simulink model "model"  (R2021a)
settings: Solver=VariableStepAuto  StartTime=0.0  StopTime=10.0  RelTol=1e-3
libraries: simulink x6, sharedutil x5, aerolibutil x1
(part 1 of 2)
settings Model: Creator=frede  LastModifiedBy=frede
settings DataIOCC: ReturnWorkspaceOutputs=off

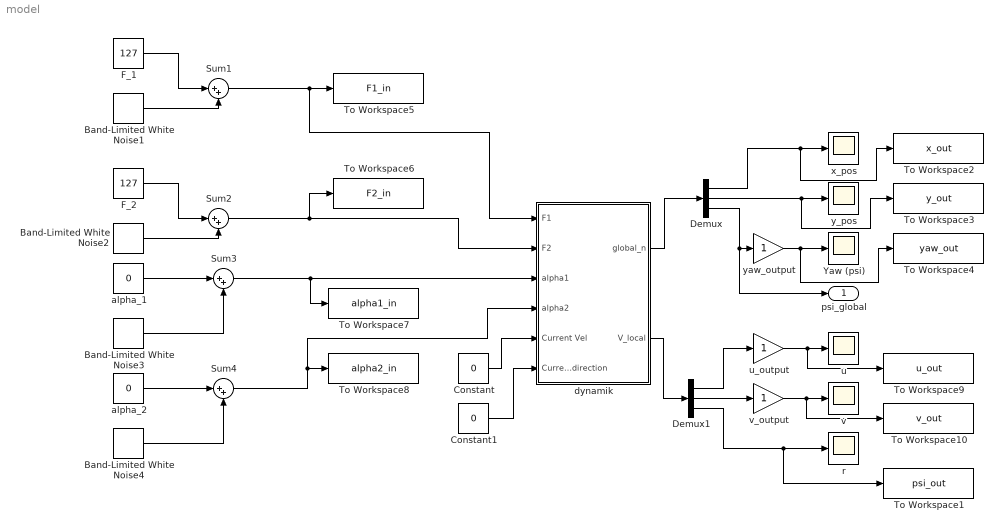
== system model ==
  Band-Limited White Noise{1..4} (4 alike) : simulink/Sources/Band-Limited White Noise  Cov=[0.01]  Ts=0.1  seed=[23341]
  Constant : Constant  Value=0
  Constant1 : Constant  Value=0
  Demux : Demux  Outputs=3
  Demux1 : Demux  Outputs=3
  F_1 : Constant  Value=127
  F_2 : Constant  Value=127
  Sum{1..4} (4 alike) : Sum  Inputs=|++
  To Workspace1 : ToWorkspace  VariableName=psi_out  SaveFormat=Timeseries  SampleTime=-1
  To Workspace10 : ToWorkspace  VariableName=v_out  SaveFormat=Timeseries  SampleTime=-1
  To Workspace2 : ToWorkspace  VariableName=x_out  SaveFormat=Timeseries  SampleTime=-1
  To Workspace3 : ToWorkspace  VariableName=y_out  SaveFormat=Timeseries  SampleTime=-1
  To Workspace4 : ToWorkspace  VariableName=yaw_out  SaveFormat=Timeseries  SampleTime=-1
  To Workspace5 : ToWorkspace  VariableName=F1_in  SaveFormat=Timeseries  SampleTime=-1
  To Workspace6 : ToWorkspace  VariableName=F2_in  SaveFormat=Timeseries  SampleTime=-1
  To Workspace7 : ToWorkspace  VariableName=alpha1_in  SaveFormat=Timeseries  SampleTime=-1
  To Workspace8 : ToWorkspace  VariableName=alpha2_in  SaveFormat=Timeseries  SampleTime=-1
  To Workspace9 : ToWorkspace  VariableName=u_out  SaveFormat=Timeseries  SampleTime=-1
  Yaw (psi) : Scope
  alpha_1 : Constant  Value=0
  alpha_2 : Constant  Value=0
  dynamik : Subsystem
  r : Scope
  u : Scope
  u_output : Gain
  v : Scope
  v_output : Gain
  x_pos : Scope
  y_pos : Scope
  yaw_output : Gain
  psi_global : Outport
  wires:
  Demux/2 -> To Workspace3/1, y_pos/1
  u_output/1 -> To Workspace9/1, u/1
  dynamik/2(V_local) -> Demux1/1
  v_output/1 -> To Workspace10/1, v/1
  Demux1/3 -> To Workspace1/1, r/1
  Demux/3 -> yaw_output/1, psi_global/1
  Demux1/1 -> u_output/1
  yaw_output/1 -> To Workspace4/1, Yaw (psi)/1
  Demux1/2 -> v_output/1
  dynamik/1(global_n) -> Demux/1
  Demux/1 -> To Workspace2/1, x_pos/1
  Constant/1 -> dynamik/5(Current Vel)
  Constant1/1 -> dynamik/6(Current direction)
  Sum3/1 -> To Workspace7/1, dynamik/3(alpha1)
  Sum4/1 -> dynamik/4(alpha2), To Workspace8/1
  Sum2/1 -> dynamik/2(F2), To Workspace6/1
  Sum1/1 -> dynamik/1(F1), To Workspace5/1
  F_1/1 -> Sum1/1
  Band-Limited White Noise1/1 -> Sum1/2
  F_2/1 -> Sum2/1
  Band-Limited White Noise2/1 -> Sum2/2
  alpha_1/1 -> Sum3/1
  Band-Limited White Noise3/1 -> Sum3/2
  Band-Limited White Noise4/1 -> Sum4/2
  alpha_2/1 -> Sum4/1

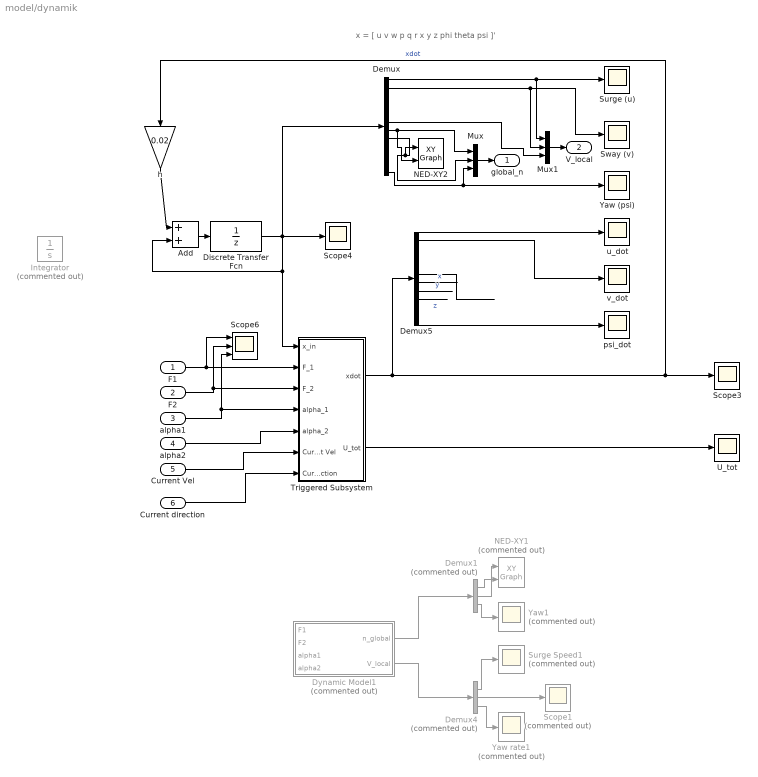
== system model/dynamik ==
  note: x = [ u v w p q r x y z phi theta psi ]'
  F1 : Inport
  F2 : Inport  Port=2
  alpha1 : Inport  Port=3
  alpha2 : Inport  Port=4
  Current Vel : Inport  Port=5
  Current direction : Inport  Port=6
  Add : Sum
  Demux : Demux  Outputs=12
  Demux1 : Demux  Commented=on  Outputs=3
  Demux4 : Demux  Commented=on  Outputs=3
  Demux5 : Demux  Outputs=12
  Discrete Transfer Fcn : DiscreteTransferFcn  Denominator=[ 1 0]  SampleTime=0.02
  Dynamic Model1 : Subsystem  Commented=on
  Integrator : Integrator  Commented=on
  Mux : Mux  Inputs=3
  Mux1 : Mux  Inputs=3
  NED-XY1 : simulink/Sinks/XY Graph  Commented=on  xmin=-1000  xmax=1000  ymin=-1000  ymax=1000  st=-1
  NED-XY2 : simulink/Sinks/XY Graph  xmin=-1000  xmax=1000  ymin=-1000  ymax=1000  st=-1
  Scope1 : Scope  Commented=on
  Scope3 : Scope
  Scope4 : Scope
  Scope6 : Scope  NumInputPorts=3
  Surge (u) : Scope
  Surge Speed1 : Scope  Commented=on
  Sway (v) : Scope
  Triggered Subsystem : Subsystem  TreatAsAtomicUnit=on
  U_tot : Scope
  Yaw (psi) : Scope
  Yaw rate1 : Scope  Commented=on
  Yaw1 : Scope  Commented=on
  h : Gain  Gain=0.02
  psi_dot : Scope
  u_dot : Scope
  v_dot : Scope
  global_n : Outport
  V_local : Outport  Port=2
  wires:
  Demux1/3 -> Yaw1/1
  Demux4/3 -> Yaw rate1/1
  Demux1/2 -> NED-XY1/1
  Demux4/2 -> Scope1/1
  Demux1/1 -> NED-XY1/2
  Demux4/1 -> Surge Speed1/1
  Dynamic Model1/1(n_global) -> Demux1/1
  Dynamic Model1/2(V_local) -> Demux4/1
  F1/1 -> Scope6/1, Triggered Subsystem/2(F_1)
  F2/1 -> Scope6/2, Triggered Subsystem/3(F_2)
  alpha1/1 -> Scope6/3, Triggered Subsystem/4(alpha_1)
  alpha2/1 -> Triggered Subsystem/5(alpha_2)
  h/1 -> Add/1
  Add/1 -> Discrete Transfer Fcn/1
  Triggered Subsystem/1(xdot) -> Demux5/1, Scope3/1, h/1  "xdot"
  Triggered Subsystem/2(U_tot) -> U_tot/1
  Demux/8 -> Mux/2, NED-XY2/1
  Demux/7 -> NED-XY2/2, Mux/1
  Discrete Transfer Fcn/1 -> Scope4/1, Demux/1, Add/2, Triggered Subsystem/1(x_in)
  Demux/1 -> Surge (u)/1, Mux1/1
  Demux/12 -> Mux/3, Yaw (psi)/1
  Demux/2 -> Mux1/2, Sway (v)/1
  Mux/1 -> global_n/1
  Demux5/12 -> psi_dot/1
  Demux5/2 -> v_dot/1
  Demux5/1 -> u_dot/1
  Demux5/9 -> ?  "z"
  Demux5/7 -> ?  "x"
  Demux5/8 -> ?  "y"
  Mux1/1 -> V_local/1
  Demux5/6 -> ?
  Demux/6 -> Mux1/3
  Current Vel/1 -> Triggered Subsystem/6(Current Vel)
  Current direction/1 -> Triggered Subsystem/7(Current Direction)

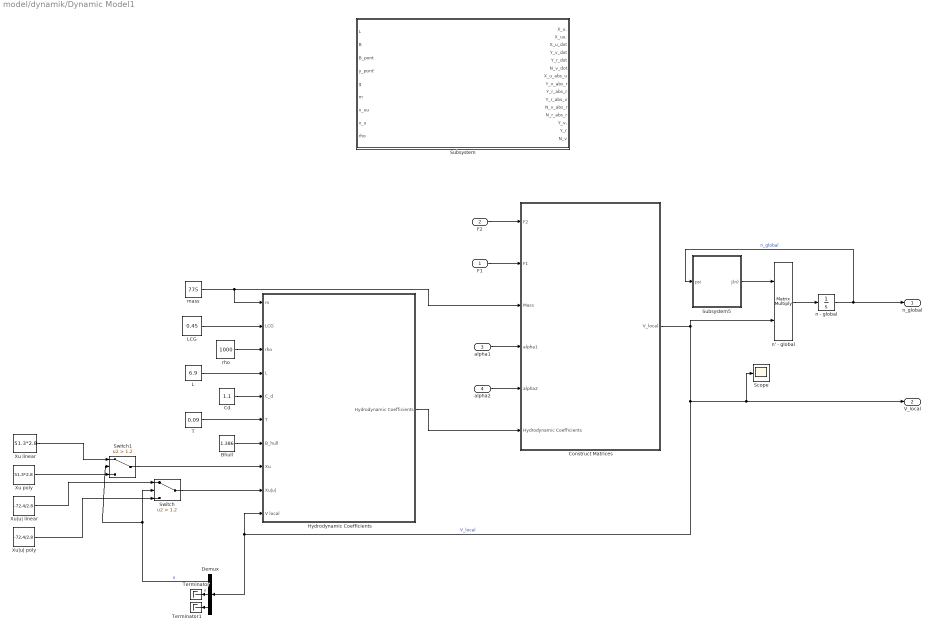
== system model/dynamik/Dynamic Model1 ==
  F1 : Inport
  F2 : Inport  Port=2
  alpha1 : Inport  Port=3
  alpha2 : Inport  Port=4
  "Bhull " : Constant  Value=1.386
  Cd : Constant  Value=1.1
  Construct Matrices : Subsystem
  Demux : Demux  Outputs=3
  Hydrodynamic Coefficients : Subsystem
  L : Constant  Value=6.9
  LCG : Constant  Value=0.45
  Scope : Scope
  Subsystem : Subsystem
  Subsystem5 : Subsystem
  Switch : Switch  Criteria=u2 > Threshold  Threshold=1.2
  Switch1 : Switch  Criteria=u2 > Threshold  Threshold=1.2
  T : Constant  Value=0.09
  Terminator : Terminator
  Terminator1 : Terminator
  Xu linear : Constant  Value=51.3*2.8
  Xu poly : Constant  Value=51.3*2.8
  Xu|u| linear : Constant  Value=-72.4/2.8
  Xu|u| poly : Constant  Value=-72.4/2.8
  mass : Constant  Value=775
  n - global : Integrator  InitialCondition=[0 0 0]
  n' - global : Product  Multiplication=Matrix(*)
  rho : Constant  Value=1000
  n_global : Outport  VectorParamsAs1DForOutWhenUnconnected=off
  V_local : Outport  Port=2  VectorParamsAs1DForOutWhenUnconnected=off
  wires:
  n - global/1 -> Subsystem5/1(psi), n_global/1  "n_global"
  Cd/1 -> Hydrodynamic Coefficients/5(C_d)
  Construct Matrices/1(V_local) -> n' - global/2, Demux/1, Hydrodynamic Coefficients/10(V local), Scope/1, V_local/1  "V_local"
  n' - global/1 -> n - global/1
  Subsystem5/1(J(n)) -> n' - global/1
  rho/1 -> Hydrodynamic Coefficients/3(rho)
  L/1 -> Hydrodynamic Coefficients/4(L)
  F2/1 -> Construct Matrices/1(F2)
  F1/1 -> Construct Matrices/2(F1)
  mass/1 -> Hydrodynamic Coefficients/1(m), Construct Matrices/3("Mass ")
  Hydrodynamic Coefficients/1("Hydrodynamic Coefficients ") -> Construct Matrices/6(Hydrodynamic Coefficients)
  T/1 -> Hydrodynamic Coefficients/6(T)
  "Bhull "/1 -> Hydrodynamic Coefficients/7(B_hull)
  Switch/1 -> Hydrodynamic Coefficients/9(Xu|u|)
  LCG/1 -> Hydrodynamic Coefficients/2(LCG)
  Demux/1 -> Switch1/2, Switch/2  "u"
  Xu|u| poly/1 -> Switch/3
  Xu|u| linear/1 -> Switch/1
  Switch1/1 -> Hydrodynamic Coefficients/8(Xu)
  Xu poly/1 -> Switch1/3
  Xu linear/1 -> Switch1/1
  Demux/3 -> Terminator1/1
  Demux/2 -> Terminator/1  "v"
  alpha1/1 -> Construct Matrices/4(alpha1)
  alpha2/1 -> Construct Matrices/5(alpha2)

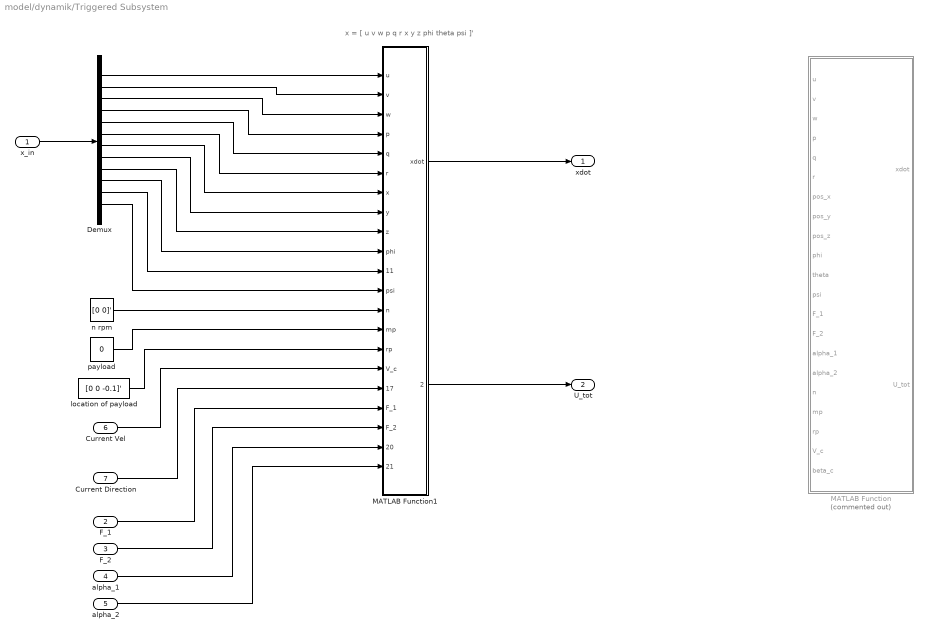
== system model/dynamik/Triggered Subsystem ==
  note: x = [ u v w p q r x y z phi theta psi ]'
  x_in : Inport
  F_1 : Inport  Port=2
  F_2 : Inport  Port=3
  alpha_1 : Inport  Port=4
  alpha_2 : Inport  Port=5
  Current Vel : Inport  Port=6
  Current Direction : Inport  Port=7
  Demux : Demux  Outputs=12
  MATLAB Function : MATLAB Function  Commented=on  TreatAsAtomicUnit=on
  MATLAB Function1 : MATLAB Function  TreatAsAtomicUnit=on
  location of payload : Constant  Value=[0 0 -0.1]'
  n rpm : Constant  Value=[0 0]'
  payload : Constant  Value=0
  xdot : Outport
  U_tot : Outport  Port=2
  wires:
  F_1/1 -> MATLAB Function1/18(F_1)
  F_2/1 -> MATLAB Function1/19(F_2)
  alpha_1/1 -> MATLAB Function1/20(alpha_1)
  alpha_2/1 -> MATLAB Function1/21(alpha_2)
  location of payload/1 -> MATLAB Function1/15(rp)
  payload/1 -> MATLAB Function1/14(mp)
  Current Vel/1 -> MATLAB Function1/16(V_c)
  Current Direction/1 -> MATLAB Function1/17(beta_c)
  n rpm/1 -> MATLAB Function1/13(n)
  x_in/1 -> Demux/1
  MATLAB Function1/2(U_tot) -> U_tot/1
  MATLAB Function1/1(xdot) -> xdot/1
  Demux/1 -> MATLAB Function1/1(u)
  Demux/2 -> MATLAB Function1/2(v)
  Demux/3 -> MATLAB Function1/3(w)
  Demux/4 -> MATLAB Function1/4(p)
  Demux/5 -> MATLAB Function1/5(q)
  Demux/6 -> MATLAB Function1/6(r)
  Demux/7 -> MATLAB Function1/7(x)
  Demux/8 -> MATLAB Function1/8(y)
  Demux/9 -> MATLAB Function1/9(z)
  Demux/10 -> MATLAB Function1/10(phi)
  Demux/11 -> MATLAB Function1/11(theta)
  Demux/12 -> MATLAB Function1/12(psi)

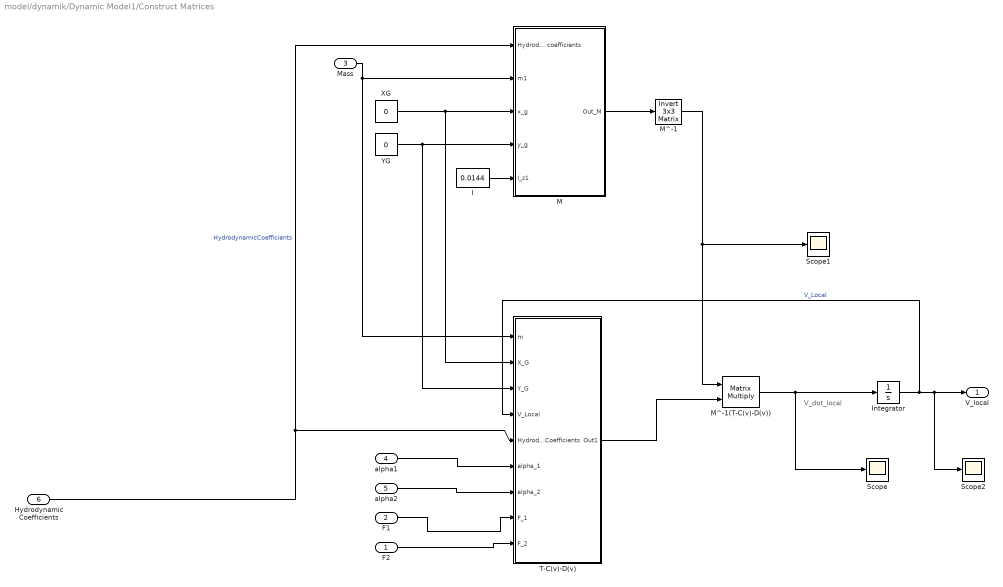
== system model/dynamik/Dynamic Model1/Construct Matrices ==
  note: V_dot_local
  F2 : Inport
  F1 : Inport  Port=2
  "Mass " : Inport  Port=3
  alpha1 : Inport  Port=4
  alpha2 : Inport  Port=5
  Hydrodynamic Coefficients : Inport  Port=6
  I : Constant  Value=0.0144
  Integrator : Integrator  InitialCondition=[0 0 0]
  M : Subsystem
  M^-1 : aerolibutil/Invert  3x3 Matrix
  M^-1(T-C(v)-D(v)) : Product  Multiplication=Matrix(*)
  Scope : Scope
  Scope1 : Scope
  Scope2 : Scope
  T-C(v)-D(v) : Subsystem
  XG : Constant  Value=0
  YG : Constant  Value=0
  V_local : Outport  VectorParamsAs1DForOutWhenUnconnected=off
  wires:
  Integrator/1 -> Scope2/1, V_local/1, T-C(v)-D(v)/4(V_Local)  "V_Local"
  M^-1(T-C(v)-D(v))/1 -> Scope/1, Integrator/1
  M/1(Out_M) -> M^-1/1
  Hydrodynamic Coefficients/1 -> M/1(Hydrodynamic coefficients), T-C(v)-D(v)/5(HydrodynamicCoefficients)  "HydrodynamicCoefficients"
  YG/1 -> M/4(y_g), T-C(v)-D(v)/3(Y_G)
  "Mass "/1 -> T-C(v)-D(v)/1(m), M/2(m1)
  XG/1 -> M/3(x_g), T-C(v)-D(v)/2(X_G)
  F1/1 -> T-C(v)-D(v)/8(F_1)
  F2/1 -> T-C(v)-D(v)/9(F_2)
  T-C(v)-D(v)/1(Out1) -> M^-1(T-C(v)-D(v))/2
  I/1 -> M/5(I_z1)
  alpha1/1 -> T-C(v)-D(v)/6(alpha_1)
  alpha2/1 -> T-C(v)-D(v)/7(alpha_2)
  M^-1/1 -> Scope1/1, M^-1(T-C(v)-D(v))/1

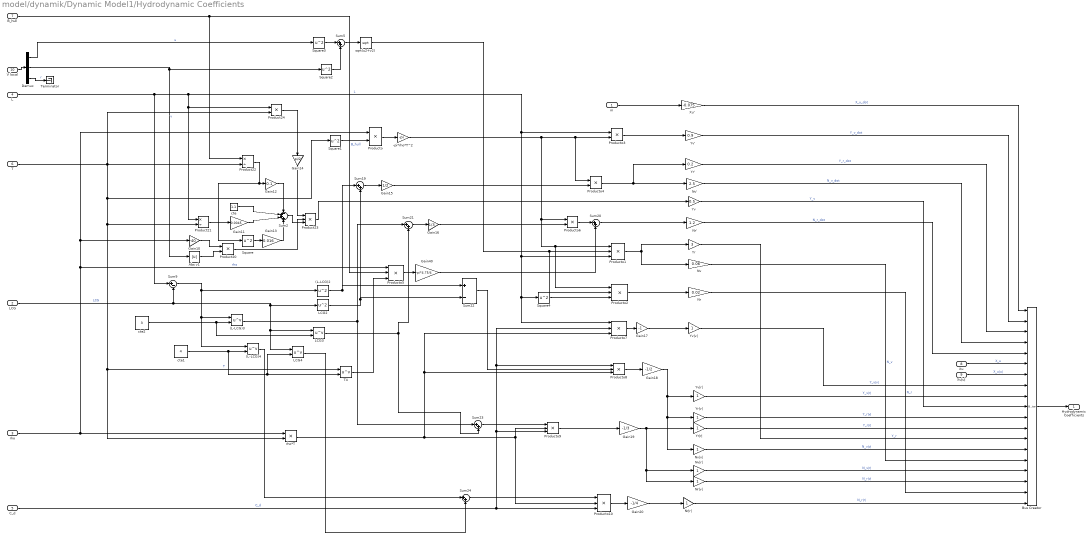
== system model/dynamik/Dynamic Model1/Hydrodynamic Coefficients ==
  m : Inport
  LCG : Inport  Port=2
  rho : Inport  Port=3
  L : Inport  Port=4
  C_d : Inport  Port=5
  T : Inport  Port=6
  B_hull : Inport  Port=7
  Xu : Inport  Port=8
  Xu|u| : Inport  Port=9
  V local : Inport  Port=10
  (L-LCG)2 : Math  Operator=square  SignedPower=on  SaturateOnIntegerOverflow=on
  (L-LCG)3 : Math  Operator=pow  SignedPower=on  SaturateOnIntegerOverflow=on
  (L-LCG)4 : Math  Operator=pow  SignedPower=on  SaturateOnIntegerOverflow=on
  -pi*rho*T^2 : Gain  Gain=-pi
  Abs v1 : Abs
  Bus Creator : BusCreator  Inputs=19
  Demux : Demux  Outputs=3
  Gain10 : Gain  Gain=-40
  Gain11 : Gain  Gain=0.0045
  Gain12 : Gain  Gain=0.1
  Gain13 : Gain  Gain=0.016
  Gain14 : Gain  Gain=pi/2
  Gain15 : Gain  Gain=1/2
  Gain16 : Gain  Gain=1/3
  Gain17 : Gain  Gain=-1
  Gain18 : Gain  Gain=-1/2
  Gain19 : Gain  Gain=-1/3
  Gain20 : Gain  Gain=-1/4
  Gain40 : Gain  Gain=-pi*4.75/4
  LCG2 : Math  Operator=square  SignedPower=on  SaturateOnIntegerOverflow=on
  LCG3 : Math  Operator=pow  SignedPower=on  SaturateOnIntegerOverflow=on
  LCG4 : Math  Operator=pow  SignedPower=on  SaturateOnIntegerOverflow=on
  Nr : Gain  Gain=0.02
  Nr' : Gain  Gain=1.2
  Nr|r| : Gain
  Nr|v| : Gain
  Nv : Gain  Gain=0.06
  Nv' : Gain  Gain=2.5
  Nv|r| : Gain
  Nv|v| : Gain
  Product20 : Product
  Product21 : Product  Inputs=*/
  Product22 : Product  Inputs=*/
  Product23 : Product  Inputs=3
  Product24 : Product
  Producto{,3..4,6} (4 alike) : Product
  Producto{1..2,5,7..10} (7 alike) : Product  Inputs=3
  Square{,1..4} (5 alike) : Math  Operator=square  SignedPower=on  SaturateOnIntegerOverflow=on
  Sum{5,19..21,23..24} (6 alike) : Sum  Inputs=|++
  Sum2 : Sum  Inputs=-+++
  Sum22 : Sum  Inputs=|+-
  Sum9 : Sum  Inputs=|+-
  T4 : Math  Operator=pow  SignedPower=on  SaturateOnIntegerOverflow=on
  Terminator : Terminator
  Xu' : Gain  Gain=-0.075
  Yr : Gain  Gain=3
  Yr' : Gain  Gain=0.2
  Yr|r| : Gain
  Yr|v| : Gain
  Yv : Gain  Gain=0.5
  Yv' : Gain  Gain=0.9
  Yv|r| : Gain
  Yv|v| : Gain
  cte : Constant  Value=1.1
  cte1 : Constant  Value=4
  cte2 : Constant  Value=3
  rho*T : Product
  sqrt(u2+v2) : Sqrt  SaturateOnIntegerOverflow=on
  "Hydrodynamic Coefficients " : Outport  VectorParamsAs1DForOutWhenUnconnected=off
  wires:
  m/1 -> Xu'/1
  Nv'/1 -> Bus Creator/4  "N_v_dot"
  Xu'/1 -> Bus Creator/1  "X_u_dot"
  Square/1 -> Gain13/1
  Gain14/1 -> Product23/1
  Product24/1 -> Gain14/1
  Sum9/1 -> (L-LCG)3/1, (L-LCG)4/1, (L-LCG)2/1
  Square4/1 -> Producto2/3
  sqrt(u2+v2)/1 -> Producto2/2, Producto1/2
  Product20/1 -> Product23/2
  Gain13/1 -> Sum2/4
  B_hull/1 -> Producto5/2, Product22/1  "B_hull"
  Square2/1 -> Sum5/2
  Sum20/1 -> Nr'/1
  Gain12/1 -> Sum2/1
  Sum21/1 -> Gain16/1
  LCG4/1 -> Sum24/2
  Sum24/1 -> Producto10/1
  (L-LCG)4/1 -> Sum24/1
  Sum2/1 -> Product23/3
  Producto10/1 -> Gain20/1
  (L-LCG)3/1 -> Sum21/1, Sum23/1
  Producto6/1 -> Sum20/1
  Gain19/1 -> Yr|r|/1, Nr|v|/1, Nv|r|/1
  Gain16/1 -> Producto6/2
  Sum22/1 -> Producto8/2
  Producto3/1 -> Yv'/1
  Gain10/1 -> Product20/1
  cte1/1 -> LCG4/2, T4/2, (L-LCG)4/2
  cte2/1 -> (L-LCG)3/2, LCG3/2
  Product23/1 -> Yv/1
  cte/1 -> Sum2/2
  Producto8/1 -> Gain18/1
  Sum23/1 -> Producto9/1
  Gain20/1 -> Nr|r|/1
  Gain18/1 -> Nv|v|/1, Yr|v|/1, Yv|r|/1
  Yr'/1 -> Bus Creator/3  "Y_r_dot"
  Producto7/1 -> Gain17/1
  Producto9/1 -> Gain19/1
  Gain11/1 -> Sum2/3
  Square1/1 -> Producto/2
  Producto2/1 -> Nr/1
  LCG3/1 -> Sum21/2, Sum23/2
  T4/1 -> Producto5/3
  Gain40/1 -> Sum20/2
  Producto4/1 -> Yr'/1, Nv'/1
  Sum19/1 -> Gain15/1
  Square3/1 -> Sum5/1
  Sum5/1 -> sqrt(u2+v2)/1
  rho/1 -> Producto/1, Gain10/1, Producto5/1, rho*T/1  "rho"
  Abs v1/1 -> Product20/2
  Product21/1 -> Gain11/1
  Gain17/1 -> Yv|v|/1
  (L-LCG)2/1 -> Sum19/1, Sum22/1
  Producto1/1 -> Nv/1, Yr/1
  Product22/1 -> Square/1, Gain12/1
  LCG2/1 -> Sum19/2, Sum22/2
  LCG/1 -> Sum9/2, LCG2/1, LCG3/1, LCG4/1  "LCG"
  Producto/1 -> -pi*rho*T^2/1
  -pi*rho*T^2/1 -> Producto4/1, Producto3/2, Producto2/1, Producto1/1, Producto6/1
  Producto5/1 -> Gain40/1
  Gain15/1 -> Producto4/2
  rho*T/1 -> Producto9/2, Producto10/2, Producto7/3, Producto8/3
  T/1 -> Product21/2, rho*T/2, T4/1, Square1/1, Product22/2, Product24/2  "T"
  L/1 -> Producto7/1, Square4/1, Producto1/3, Producto3/1, Product21/1, Product24/1, Sum9/1  "L"
  C_d/1 -> Producto7/2, Producto8/1, Producto9/3, Producto10/3  "C_d"
  Nv/1 -> Bus Creator/15  "N_v"
  Yv|v|/1 -> Bus Creator/8  "Y_v|v|"
  Yr|r|/1 -> Bus Creator/12  "Y_r|r|"
  Yv/1 -> Bus Creator/10  "Y_v"
  Nv|v|/1 -> Bus Creator/14  "N_v|v|"
  Yr|v|/1 -> Bus Creator/11  "Y_r|v|"
  Nv|r|/1 -> Bus Creator/16  "N_v|r|"
  Yr/1 -> Bus Creator/13  "Y_r"
  Nr|r|/1 -> Bus Creator/19  "N_r|r|"
  Nr/1 -> Bus Creator/18  "N_r"
  Xu|u|/1 -> Bus Creator/7  "X_u|u|"
  Yv|r|/1 -> Bus Creator/9  "Y_v|r|"
  Nr|v|/1 -> Bus Creator/17  "N_r|v|"
  Xu/1 -> Bus Creator/6  "X_u"
  Bus Creator/1 -> "Hydrodynamic Coefficients "/1
  Nr'/1 -> Bus Creator/5  "N_r_dot"
  Yv'/1 -> Bus Creator/2  "Y_v_dot"
  Demux/1 -> Square3/1  "u"
  V local/1 -> Demux/1
  Demux/2 -> Abs v1/1, Square2/1  "v"
  Demux/3 -> Terminator/1  "r"

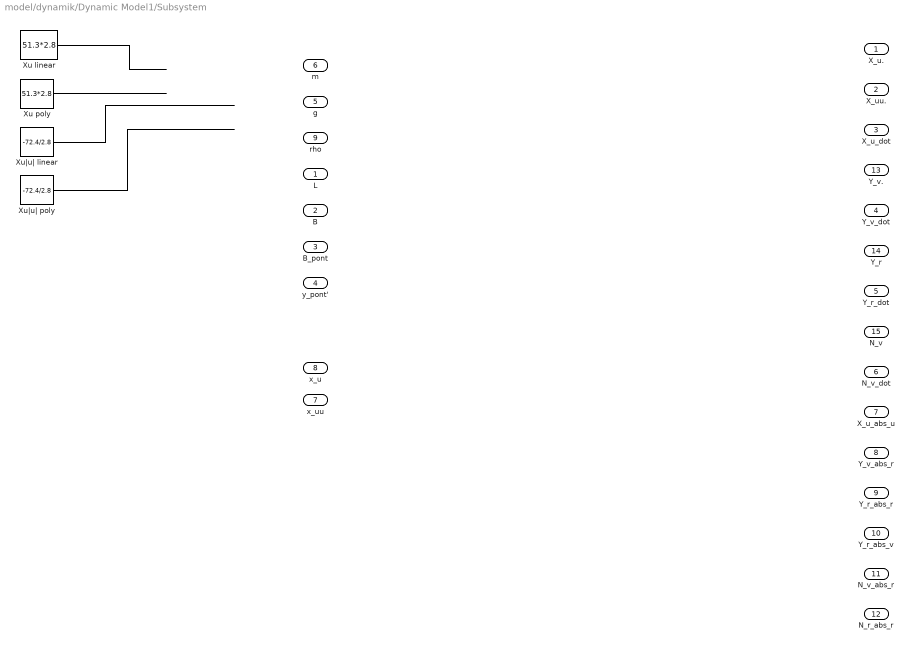
== system model/dynamik/Dynamic Model1/Subsystem ==
  L : Inport
  B : Inport  Port=2
  B_pont : Inport  Port=3
  y_pont' : Inport  Port=4
  g : Inport  Port=5
  m : Inport  Port=6
  x_uu : Inport  Port=7
  x_u : Inport  Port=8
  rho : Inport  Port=9
  Xu linear : Constant  Value=51.3*2.8
  Xu poly : Constant  Value=51.3*2.8
  Xu|u| linear : Constant  Value=-72.4/2.8
  Xu|u| poly : Constant  Value=-72.4/2.8
  X_u. : Outport
  X_uu. : Outport  Port=2
  X_u_dot : Outport  Port=3
  Y_v_dot : Outport  Port=4
  Y_r_dot : Outport  Port=5
  N_v_dot : Outport  Port=6
  X_u_abs_u : Outport  Port=7
  Y_v_abs_r : Outport  Port=8
  Y_r_abs_r : Outport  Port=9
  Y_r_abs_v : Outport  Port=10
  N_v_abs_r : Outport  Port=11
  N_r_abs_r : Outport  Port=12
  Y_v. : Outport  Port=13
  Y_r : Outport  Port=14
  N_v : Outport  Port=15
  wires:
  Xu|u| linear/1 -> ?
  Xu|u| poly/1 -> ?
  Xu poly/1 -> ?
  Xu linear/1 -> ?

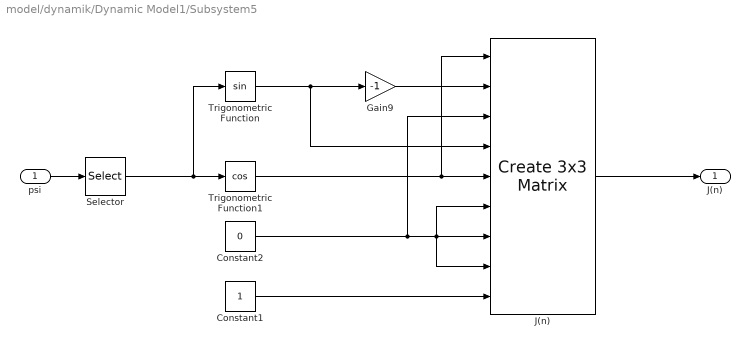
== system model/dynamik/Dynamic Model1/Subsystem5 ==
  psi : Inport
  " J(n)" : sharedutil/Create 3x3 Matrix  aMode=aMode
      settings: SourceProductBaseCode=AE,PW,DR,MT,UV,VE
  Constant1 : Constant
  Constant2 : Constant  Value=0
  Gain9 : Gain  Gain=-1
  Selector : Selector  InputPortWidth=3  IndexOptions=Index vector (dialog)  Indices=3  OutputSizes=1
  Trigonometric Function : Trigonometry
  Trigonometric Function1 : Trigonometry  Operator=cos
  J(n) : Outport  VectorParamsAs1DForOutWhenUnconnected=off
  wires:
  Gain9/1 -> " J(n)"/2
  Trigonometric Function1/1 -> " J(n)"/5, " J(n)"/1
  Trigonometric Function/1 -> " J(n)"/4, Gain9/1
  Constant1/1 -> " J(n)"/9
  psi/1 -> Selector/1
  " J(n)"/1 -> J(n)/1
  Constant2/1 -> " J(n)"/8, " J(n)"/7, " J(n)"/6, " J(n)"/3
  Selector/1 -> Trigonometric Function1/1, Trigonometric Function/1

== system model/dynamik/Dynamic Model1/Construct Matrices/M ==
  Hydrodynamic coefficients : Inport
  m1 : Inport  Port=2
  x_g : Inport  Port=3
  y_g : Inport  Port=4
  I_z1 : Inport  Port=5
  Bus Selector : BusSelector  OutputSignals=X_u_dot,Y_r_dot,N_v_dot,Y_v_dot,N_r_dot
  M-matrice : MATLAB Function  TreatAsAtomicUnit=on
  Out_M : Outport
  wires:
  Hydrodynamic coefficients/1 -> Bus Selector/1
  m1/1 -> M-matrice/1(m)
  I_z1/1 -> M-matrice/4(I_z)
  y_g/1 -> M-matrice/3(y_g)
  x_g/1 -> M-matrice/2(x_g)
  M-matrice/1(M_out) -> Out_M/1
  Bus Selector/1 -> M-matrice/5(Xu_dot)  "<X_u_dot>"
  Bus Selector/2 -> M-matrice/7(Yr_dot)  "<Y_r_dot>"
  Bus Selector/4 -> M-matrice/6(Yv_dot)  "<Y_v_dot>"
  Bus Selector/5 -> M-matrice/8(Nr_dot)  "<N_r_dot>"
  Bus Selector/3 -> M-matrice/9(Nv_dot)  "<N_v_dot>"

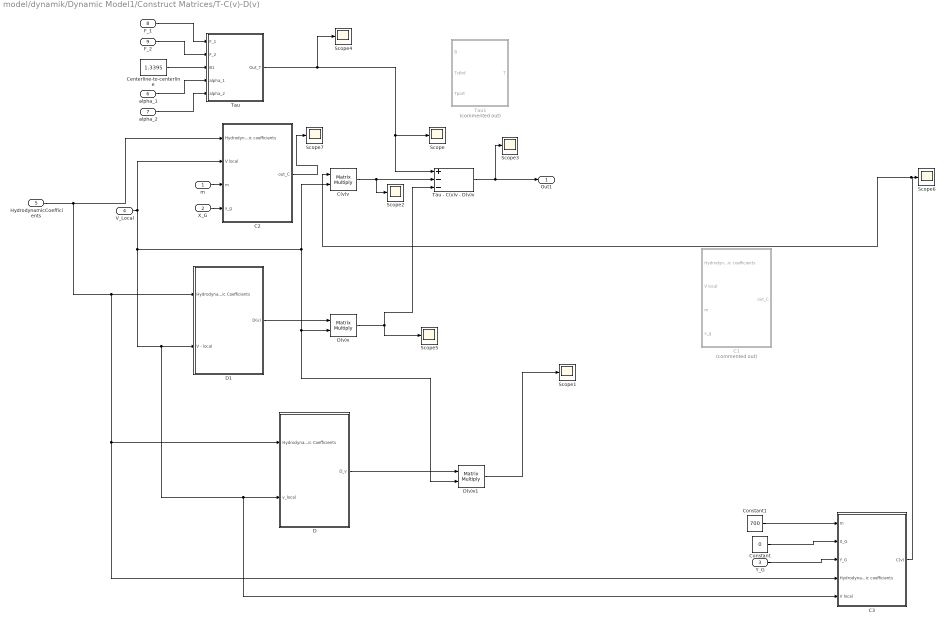
== system model/dynamik/Dynamic Model1/Construct Matrices/T-C(v)-D(v) ==
  m : Inport
  X_G : Inport  Port=2
  Y_G : Inport  Port=3
  V_Local : Inport  Port=4
  HydrodynamicCoefficients : Inport  Port=5
  alpha_1 : Inport  Port=6
  alpha_2 : Inport  Port=7
  F_1 : Inport  Port=8
  F_2 : Inport  Port=9
  C(v)v : Product  Multiplication=Matrix(*)
  C1 : Subsystem  Commented=on
  C2 : Subsystem
  C3 : Subsystem
  Centerline-to-centerline : Constant  Value=1.3395
  Constant : Constant  Value=0
  Constant1 : Constant  Value=700
  D : Subsystem
  D(v)v : Product  Multiplication=Matrix(*)
  D(v)v1 : Product  Multiplication=Matrix(*)
  D1 : Subsystem
  Scope{,1..7} (8 alike) : Scope
  Tau : Subsystem
  Tau - C(v)v - D(v)v : Sum  Inputs=+--
  Tau1 : Subsystem  Commented=on
  Out1 : Outport  VectorParamsAs1DForOutWhenUnconnected=off
  wires:
  V_Local/1 -> C2/2(V local), C3/5(V local), D/2(v_local), D1/2(V - local), D(v)v1/2, D(v)v/2, C(v)v/2
  Tau - C(v)v - D(v)v/1 -> Scope3/1, Out1/1
  HydrodynamicCoefficients/1 -> C2/1(Hydrodynamic coefficients), D/1(Hydrodynamic Coefficients), C3/4(Hydrodynamic coefficients), D1/1(Hydrodynamic Coefficients)
  Centerline-to-centerline/1 -> Tau/3(B1)
  F_2/1 -> Tau/2(F_2)
  F_1/1 -> Tau/1(F_1)
  m/1 -> C2/3(m)
  X_G/1 -> C2/4(x_g)
  Y_G/1 -> C3/3(Y_G)
  C2/1(out_C) -> Scope7/1
  D1/1(D(v)) -> D(v)v/1
  C(v)v/1 -> Scope2/1, Tau - C(v)v - D(v)v/2
  alpha_1/1 -> Tau/4(alpha_1)
  alpha_2/1 -> Tau/5(alpha_2)
  D/1(D_v) -> D(v)v1/1
  D(v)v/1 -> Tau - C(v)v - D(v)v/3, Scope5/1
  D(v)v1/1 -> Scope1/1
  Tau/1(Out_T) -> Scope4/1, Scope/1, Tau - C(v)v - D(v)v/1
  Constant/1 -> C3/2(X_G)
  Constant1/1 -> C3/1(m)
  C3/1(C(v)) -> C(v)v/1, Scope6/1

== system model/dynamik/Dynamic Model1/Construct Matrices/T-C(v)-D(v)/C1 ==
  Hydrodynamic coefficients : Inport
  V local : Inport  Port=2
  m : Inport  Port=3
  x_g : Inport  Port=4
  Demux : Demux  Outputs=19
  Demux1 : Demux  Outputs=3
  MATLAB Function : MATLAB Function  TreatAsAtomicUnit=on
  out_C : Outport
  wires:
  Hydrodynamic coefficients/1 -> Demux/1
  V local/1 -> Demux1/1
  MATLAB Function/1(y) -> out_C/1
  Demux1/1 -> MATLAB Function/2(u)  "u"
  Demux1/2 -> MATLAB Function/1(v)  "v"
  Demux1/3 -> MATLAB Function/3(r)  "r"
  Demux/1 -> MATLAB Function/6(Xu_dot)
  Demux/2 -> MATLAB Function/7(Yv_dot)
  Demux/3 -> MATLAB Function/8(Yr_dot)
  x_g/1 -> MATLAB Function/5(x_g)
  m/1 -> MATLAB Function/4(m)

== system model/dynamik/Dynamic Model1/Construct Matrices/T-C(v)-D(v)/C2 ==
  Hydrodynamic coefficients : Inport
  V local : Inport  Port=2
  m : Inport  Port=3
  x_g : Inport  Port=4
  Demux : Demux  Outputs=19
  Demux1 : Demux  Outputs=3
  MATLAB Function : MATLAB Function  TreatAsAtomicUnit=on
  out_C : Outport
  wires:
  Hydrodynamic coefficients/1 -> Demux/1
  V local/1 -> Demux1/1
  MATLAB Function/1(y) -> out_C/1
  Demux1/1 -> MATLAB Function/2(u)  "u"
  Demux1/2 -> MATLAB Function/1(v)  "v"
  Demux1/3 -> MATLAB Function/3(r)  "r"
  Demux/1 -> MATLAB Function/6(Xu_dot)
  Demux/2 -> MATLAB Function/7(Yv_dot)
  Demux/3 -> MATLAB Function/8(Yr_dot)
  x_g/1 -> MATLAB Function/5(x_g)
  m/1 -> MATLAB Function/4(m)

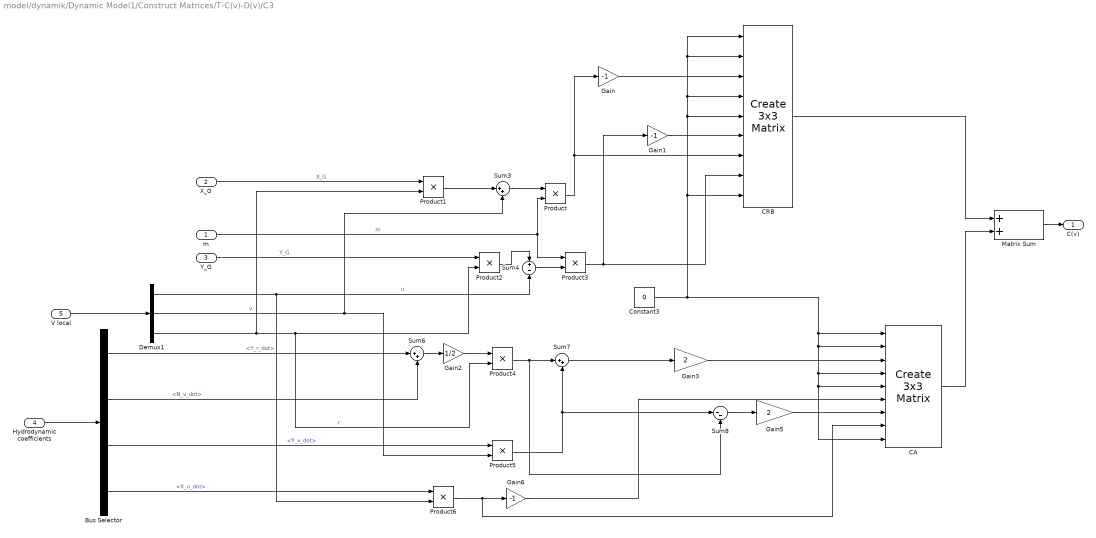
== system model/dynamik/Dynamic Model1/Construct Matrices/T-C(v)-D(v)/C3 ==
  m : Inport
  X_G : Inport  Port=2
  Y_G : Inport  Port=3
  Hydrodynamic coefficients : Inport  Port=4
  V local : Inport  Port=5
  " CRB" : sharedutil/Create 3x3 Matrix  aMode=aMode
      settings: SourceProductBaseCode=AE,PW,DR,MT,UV,VE
  Bus Selector : BusSelector  OutputSignals=Y_r_dot,N_v_dot,Y_v_dot,X_u_dot
  CA : sharedutil/Create 3x3 Matrix  aMode=aMode
      settings: SourceProductBaseCode=AE,PW,DR,MT,UV,VE
  Constant3 : Constant  Value=0
  Demux1 : Demux  Outputs=3
  Gain : Gain  Gain=-1
  Gain1 : Gain  Gain=-1
  Gain2 : Gain  Gain=1/2
  Gain3 : Gain  Gain=2
  Gain5 : Gain  Gain=2
  Gain6 : Gain  Gain=-1
  Matrix Sum : Sum
  Product{,1..6} (7 alike) : Product
  Sum3 : Sum  Inputs=|++
  Sum4 : Sum  Inputs=+-
  Sum6 : Sum  Inputs=|++
  Sum7 : Sum  Inputs=|++
  Sum8 : Sum  Inputs=|--
  C(v) : Outport  VectorParamsAs1DForOutWhenUnconnected=off
  wires:
  Bus Selector/1 -> Sum6/1  "<Y_r_dot>"
  Demux1/3 -> Product1/2, Product2/2, Product4/2  "r"
  Gain2/1 -> Product4/1
  CA/1 -> Matrix Sum/2
  Gain/1 -> " CRB"/3
  Bus Selector/2 -> Sum6/2  "<N_v_dot>"
  Sum3/1 -> Product/1
  Sum8/1 -> Gain5/1
  Product2/1 -> Sum4/1
  Sum6/1 -> Gain2/1
  Product5/1 -> Sum7/2, Sum8/1
  Gain1/1 -> " CRB"/6
  Product1/1 -> Sum3/1
  Y_G/1 -> Product2/1  "Y_G"
  Matrix Sum/1 -> C(v)/1
  Gain3/1 -> CA/3
  Gain6/1 -> CA/6
  Product6/1 -> Gain6/1, CA/8
  Demux1/2 -> Sum3/2, Product5/2  "v"
  Product4/1 -> Sum7/1, Sum8/2
  Product3/1 -> " CRB"/8, Gain1/1
  Gain5/1 -> CA/7
  " CRB"/1 -> Matrix Sum/1
  X_G/1 -> Product1/1  "X_G"
  Sum7/1 -> Gain3/1
  Product/1 -> " CRB"/7, Gain/1
  m/1 -> Product/2, Product3/1  "m"
  Constant3/1 -> " CRB"/5, " CRB"/4, " CRB"/2, " CRB"/1, " CRB"/9, CA/4, CA/5, CA/9, CA/2, CA/1
  Hydrodynamic coefficients/1 -> Bus Selector/1
  Bus Selector/4 -> Product6/1  "<X_u_dot>"
  Bus Selector/3 -> Product5/1  "<Y_v_dot>"
  Demux1/1 -> Sum4/2, Product6/2  "u"
  V local/1 -> Demux1/1
  Sum4/1 -> Product3/2

== system model/dynamik/Dynamic Model1/Construct Matrices/T-C(v)-D(v)/D ==
  Hydrodynamic Coefficients : Inport
  v_local : Inport  Port=2
  Bus Selector : BusSelector  OutputSignals=X_u,Y_v,Y_r,X_u|u|,Y_v|v|,Y_v|r|,Y_r|v|,N_v,N_r,Y_r|r|,N_v|v|,N_v|r|,N_r|r|,N_r|v|
  Demux1 : Demux  Outputs=3
  MATLAB Function : MATLAB Function  TreatAsAtomicUnit=on
  D_v : Outport
  wires:
  Hydrodynamic Coefficients/1 -> Bus Selector/1
  Demux1/3 -> MATLAB Function/3(r)
  MATLAB Function/1(D_v) -> D_v/1
  v_local/1 -> Demux1/1
  Bus Selector/1 -> MATLAB Function/4(X_u)  "<X_u>"
  Bus Selector/2 -> MATLAB Function/5(Y_v)  "<Y_v>"
  Bus Selector/14 -> MATLAB Function/16(N_r_abs_v)  "<N_r|v|>"
  Bus Selector/13 -> MATLAB Function/15(N_r_abs_r)  "<N_r|r|>"
  Bus Selector/12 -> ?  "<N_v|r|>"
  Bus Selector/11 -> MATLAB Function/14(N_v_abs_v)  "<N_v|v|>"
  Bus Selector/10 -> MATLAB Function/13(Y_r_abs_r)  "<Y_r|r|>"
  Bus Selector/9 -> MATLAB Function/7(N_r)  "<N_r>"
  Bus Selector/8 -> MATLAB Function/8(N_v)  "<N_v>"
  Bus Selector/7 -> MATLAB Function/12(Y_r_abs_v)  "<Y_r|v|>"
  Bus Selector/6 -> MATLAB Function/10(Y_v_abs_r)  "<Y_v|r|>"
  Bus Selector/5 -> MATLAB Function/9(Y_v_abs_v)  "<Y_v|v|>"
  Bus Selector/4 -> MATLAB Function/11(x_u_abs_u)  "<X_u|u|>"
  Bus Selector/3 -> MATLAB Function/6(Y_r)  "<Y_r>"
  Demux1/1 -> MATLAB Function/2(u)
  Demux1/2 -> MATLAB Function/1(v)

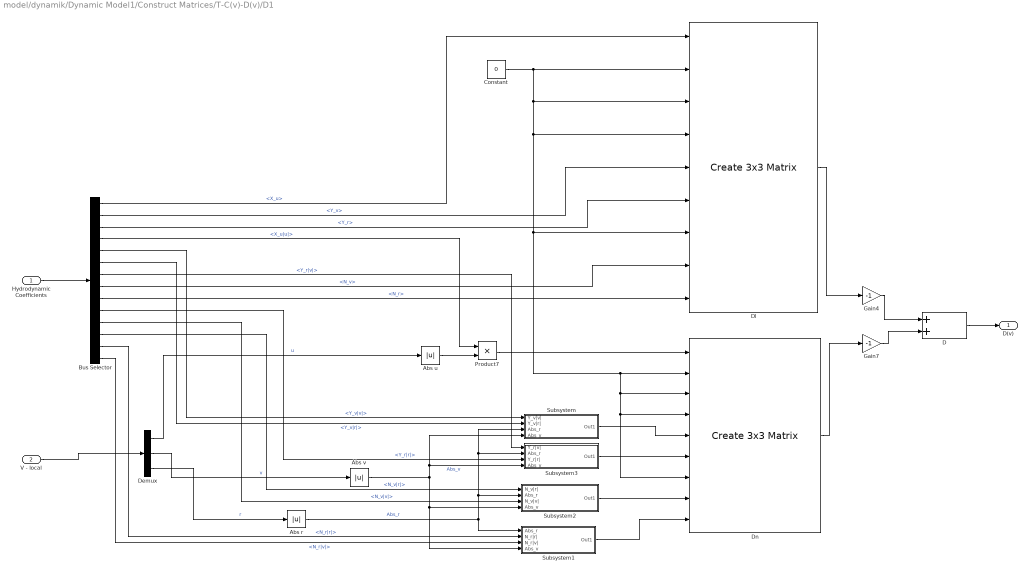
== system model/dynamik/Dynamic Model1/Construct Matrices/T-C(v)-D(v)/D1 ==
  Hydrodynamic Coefficients : Inport
  V - local : Inport  Port=2
  Abs r : Abs
  Abs u : Abs
  Abs v : Abs
  Bus Selector : BusSelector  OutputSignals=X_u,Y_v,Y_r,X_u|u|,Y_v|v|,Y_v|r|,Y_r|v|,N_v,N_r,Y_r|r|,N_v|v|,N_v|r|,N_r|r|,N_r|v|
  Constant : Constant  Value=0
  D : Sum
  Demux : Demux  Outputs=3
  Dl : sharedutil/Create 3x3 Matrix  aMode=aMode
      settings: SourceProductBaseCode=AE,PW,DR,MT,UV,VE
  Dn : sharedutil/Create 3x3 Matrix  aMode=aMode
      settings: SourceProductBaseCode=AE,PW,DR,MT,UV,VE
  Gain4 : Gain  Gain=-1
  Gain7 : Gain  Gain=-1
  Product7 : Product
  Subsystem : Subsystem
  Subsystem1 : Subsystem
  Subsystem2 : Subsystem
  Subsystem3 : Subsystem
  D(v) : Outport  VectorParamsAs1DForOutWhenUnconnected=off
  wires:
  Constant/1 -> Dn/7, Dn/4, Dn/3, Dn/2, Dl/7, Dl/4, Dl/3, Dl/2
  Abs u/1 -> Product7/2
  Abs r/1 -> Subsystem/3(Abs_r), Subsystem3/2("Abs_r "), Subsystem2/2(Abs_r), Subsystem1/1(Abs_r)  "Abs_r"
  Product7/1 -> Dn/1
  Abs v/1 -> Subsystem/4("Abs_v "), Subsystem3/4(Abs_v), Subsystem1/4(Abs_v), Subsystem2/4(Abs_v)  "Abs_v"
  Gain7/1 -> D/2
  Gain4/1 -> D/1
  Dl/1 -> Gain4/1
  Dn/1 -> Gain7/1
  D/1 -> D(v)/1
  Subsystem/1(Out1) -> Dn/5
  Subsystem1/1(Out1) -> Dn/9
  Subsystem2/1(Out1) -> Dn/8
  Subsystem3/1(Out1) -> Dn/6
  Hydrodynamic Coefficients/1 -> Bus Selector/1
  Bus Selector/5 -> Subsystem/1("Y_v|v| ")  "<Y_v|v|>"
  Bus Selector/6 -> Subsystem/2(Y_v|r|)  "<Y_v|r|>"
  Bus Selector/2 -> Dl/5  "<Y_v>"
  Bus Selector/7 -> Subsystem3/1(Y_r|v|)  "<Y_r|v|>"
  Bus Selector/10 -> Subsystem3/3(Y_r|r|)  "<Y_r|r|>"
  Bus Selector/11 -> Subsystem2/3(N_v|v|)  "<N_v|v|>"
  Bus Selector/8 -> Dl/8  "<N_v>"
  Bus Selector/12 -> Subsystem2/1(N_v|r|)  "<N_v|r|>"
  Bus Selector/14 -> Subsystem1/3(N_r|v|)  "<N_r|v|>"
  Bus Selector/9 -> Dl/9  "<N_r>"
  Bus Selector/13 -> Subsystem1/2(N_r|r|)  "<N_r|r|>"
  Bus Selector/1 -> Dl/1  "<X_u>"
  Bus Selector/4 -> Product7/1  "<X_u|u|>"
  Bus Selector/3 -> Dl/6  "<Y_r>"
  Demux/1 -> Abs u/1  "u"
  Demux/2 -> Abs v/1  "v"
  Demux/3 -> Abs r/1  "r"
  V - local/1 -> Demux/1

== system model/dynamik/Dynamic Model1/Construct Matrices/T-C(v)-D(v)/Tau ==
  F_1 : Inport
  F_2 : Inport  Port=2
  B1 : Inport  Port=3
  alpha_1 : Inport  Port=4
  alpha_2 : Inport  Port=5
  MATLAB Function : MATLAB Function  TreatAsAtomicUnit=on
  MATLAB Function1 : MATLAB Function  Commented=on  TreatAsAtomicUnit=on
  Out_T : Outport
  wires:
  F_1/1 -> MATLAB Function/1(F_1)
  MATLAB Function/1(y) -> Out_T/1
  B1/1 -> MATLAB Function/5(d)
  F_2/1 -> MATLAB Function/2(F_2)
  alpha_1/1 -> MATLAB Function/3(alpha_1)
  alpha_2/1 -> MATLAB Function/4(alpha_2)

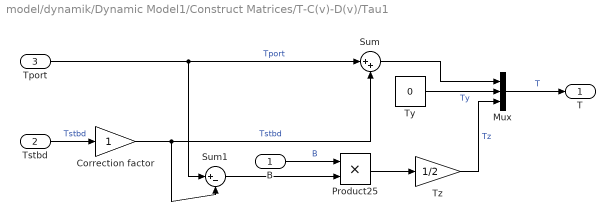
== system model/dynamik/Dynamic Model1/Construct Matrices/T-C(v)-D(v)/Tau1 ==
  B : Inport
  Tstbd : Inport  Port=2
  Tport : Inport  Port=3
  Correction factor : Gain
  Mux : Mux  Inputs=3
  Product25 : Product
  Sum : Sum  Inputs=|++
  Sum1 : Sum  Inputs=|+-
  Ty : Constant  Value=0
  Tz : Gain  Gain=1/2
  T : Outport  VectorParamsAs1DForOutWhenUnconnected=off
  wires:
  Product25/1 -> Tz/1
  Tz/1 -> Mux/3  "Tz"
  Mux/1 -> T/1  "T"
  B/1 -> Product25/1  "B"
  Sum1/1 -> Product25/2
  Ty/1 -> Mux/2  "Ty"
  Tstbd/1 -> Correction factor/1  "Tstbd"
  Tport/1 -> Sum/1, Sum1/1  "Tport"
  Sum/1 -> Mux/1
  Correction factor/1 -> Sum/2, Sum1/2  "Tstbd"

== system model/dynamik/Dynamic Model1/Construct Matrices/T-C(v)-D(v)/D1/Subsystem ==
  "Y_v|v| " : Inport
  Y_v|r| : Inport  Port=2
  Abs_r : Inport  Port=3
  "Abs_v " : Inport  Port=4
  Product8 : Product
  Product9 : Product
  Sum10 : Sum  Inputs=|++
  Out1 : Outport  VectorParamsAs1DForOutWhenUnconnected=off
  wires:
  Y_v|r|/1 -> Product9/1
  Abs_r/1 -> Product9/2
  Product9/1 -> Sum10/2
  "Y_v|v| "/1 -> Product8/1
  Product8/1 -> Sum10/1
  "Abs_v "/1 -> Product8/2
  Sum10/1 -> Out1/1

== system model/dynamik/Dynamic Model1/Construct Matrices/T-C(v)-D(v)/D1/Subsystem1 ==
  Abs_r : Inport
  N_r|r| : Inport  Port=2
  N_r|v| : Inport  Port=3
  Abs_v : Inport  Port=4
  Product14 : Product
  Product15 : Product
  Sum13 : Sum  Inputs=|++
  Out1 : Outport  VectorParamsAs1DForOutWhenUnconnected=off
  wires:
  Product15/1 -> Sum13/1
  Sum13/1 -> Out1/1
  N_r|v|/1 -> Product14/1
  Product14/1 -> Sum13/2
  Abs_r/1 -> Product15/2
  N_r|r|/1 -> Product15/1
  Abs_v/1 -> Product14/2

== system model/dynamik/Dynamic Model1/Construct Matrices/T-C(v)-D(v)/D1/Subsystem2 ==
  N_v|r| : Inport
  Abs_r : Inport  Port=2
  N_v|v| : Inport  Port=3
  Abs_v : Inport  Port=4
  Product12 : Product
  Product13 : Product
  Sum12 : Sum  Inputs=|++
  Out1 : Outport  VectorParamsAs1DForOutWhenUnconnected=off
  wires:
  Sum12/1 -> Out1/1
  Product13/1 -> Sum12/1
  N_v|v|/1 -> Product12/1
  Product12/1 -> Sum12/2
  Abs_r/1 -> Product13/2
  Abs_v/1 -> Product12/2
  N_v|r|/1 -> Product13/1

== system model/dynamik/Dynamic Model1/Construct Matrices/T-C(v)-D(v)/D1/Subsystem3 ==
  Y_r|v| : Inport
  "Abs_r " : Inport  Port=2
  Y_r|r| : Inport  Port=3
  Abs_v : Inport  Port=4
  Product10 : Product
  Product11 : Product
  Sum11 : Sum  Inputs=|++
  Out1 : Outport  VectorParamsAs1DForOutWhenUnconnected=off
  wires:
  Product11/1 -> Sum11/2
  Product10/1 -> Sum11/1
  Sum11/1 -> Out1/1
  Y_r|v|/1 -> Product10/1
  "Abs_r "/1 -> Product11/2
  Y_r|r|/1 -> Product11/1
  Abs_v/1 -> Product10/2

== matlab function model/dynamik/Dynamic Model1/Construct Matrices/T-C(v)-D(v)/C1/MATLAB Function ==
  data: v input; u input; r input; y output; m input; x_g input; Xu_dot input; Yv_dot input; Yr_dot input
function y = fcn(v, u,r, m,x_g, Xu_dot, Yv_dot, Yr_dot)

    
    C_RB = [    0       ,     0     , -m*(x_g*r+v);
                0       ,     0     ,      m*u    ;
            m*(x_g*r+v) ,   -m*u    ,       0     ]



    C_A = [           0      ,     0     , Yv_dot*v+Yr_dot*r;
                      0      ,     0     ,     -Xu_dot*u    ;
            -Yv_dot*v-Yr_dot ,  Xu_dot*u ,         0        ]


    C = C_A + C_RB









y = C;

== matlab function model/dynamik/Dynamic Model1/Construct Matrices/T-C(v)-D(v)/C2/MATLAB Function ==
  data: v input; u input; r input; y output; m input; x_g input; Xu_dot input; Yv_dot input; Yr_dot input
function y = fcn(v, u,r, m,x_g, Xu_dot, Yv_dot, Yr_dot)

    
    C_RB = [    0       ,     0     , -m*(x_g*r+v);
                0       ,     0     ,      m*u    ;
            m*(x_g*r+v) ,   -m*u    ,       0     ]



    C_A = [           0      ,     0     , Yv_dot*v+Yr_dot*r;
                      0      ,     0     ,     -Xu_dot*u    ;
            -Yv_dot*v-Yr_dot ,  Xu_dot*u ,         0        ]


    C = C_A + C_RB









y = C;

== matlab function model/dynamik/Dynamic Model1/Construct Matrices/T-C(v)-D(v)/D/MATLAB Function ==
  data: v input; u input; r input; X_u input; D_v output; Y_v input; Y_r input; N_r input; N_v input; Y_v_abs_v input; Y_v_abs_r input; x_u_abs_u input; Y_r_abs_v input; Y_r_abs_r input; N_v_abs_v input; N_r_abs_r input; N_r_abs_v input
function D_v = fcn(v,u,r, X_u, Y_v, Y_r, N_r, N_v, Y_v_abs_v, Y_v_abs_r, x_u_abs_u, Y_r_abs_v, Y_r_abs_r, N_v_abs_v, N_r_abs_r, N_r_abs_v)
    %v = v_(1);
    %u = v_(2);
    %r = v_(3);


    D_RB = [-X_u ,   0  ,  0 ;
              0  , -Y_v , -Y_r;
             0   , -N_v , -N_r];
                
                  
    D_A = [-(x_u_abs_u)*abs(u)   ,                 0                          ,                         0                 ;
                      0          , -(Y_v_abs_v)*(abs(v))+(Y_v_abs_r)*(abs(r)) , -((Y_r_abs_v)*(abs(v))+(Y_r_abs_r)*(abs(r)));
                      0          , -(N_v_abs_v)*(abs(v))+(Y_v_abs_r)*(abs(r)) , -((N_r_abs_v)*(abs(v))+(N_r_abs_r)*(abs(r)))];
        
        

    D = D_RB + D_A;


D_v = D;

== matlab function model/dynamik/Dynamic Model1/Construct Matrices/T-C(v)-D(v)/Tau/MATLAB Function ==
  data: F_1 input; y output; F_2 input; alpha_1 input; alpha_2 input; d input
function y = fcn(F_1, F_2, alpha_1, alpha_2, d)
  
    % tau = [tau_x ; tau_y ; tau_z];
% 
%     force = [  F_1*cos(alpha_1)+F_2*cos(alpha_2)   ;
%                F_1*sin(alpha_1)+F_2*sin(alpha_2)   ;
%              F_1*d*cos(alpha_1)-F_2*d*cos(alpha_2)];
    
    force = [  F_1*cos(alpha_1)+F_2*cos(alpha_2)   ;
               F_1*sin(alpha_1)+F_2*sin(alpha_2)   ;
             F_1*d*cos(alpha_1)-F_2*d*cos(alpha_2)];     
    
y = force;

== matlab function model/dynamik/Dynamic Model1/Construct Matrices/T-C(v)-D(v)/Tau/MATLAB Function1 ==
  data: T_stbd input; y output; T_port input; B input
function y = fcn(T_stbd, T_port, B)
  
    % tau = [tau_x ; tau_y ; tau_z];

    tau = [   T_port + T_stbd   ;
                     0          ;
           (B*(T_port-T_stbd)/2)];
y = tau;

== matlab function model/dynamik/Triggered Subsystem/MATLAB Function ==
  settings: updateMethod=DISCRETE
  data: xdot output; U_tot output; u input; v input; w input; p input; q input; r input; pos_x input; pos_y input; pos_z input; phi input; theta input; psi input; F_1 input; F_2 input; alpha_1 input; alpha_2 input; n input; mp input; rp input; V_c input; beta_c input
function [xdot, U_tot]  = otter(u, v, w, p, q, r, pos_x, pos_y, pos_z, phi, theta, psi ,F_1,F_2,alpha_1,alpha_2,n,mp,rp,V_c,beta_c)
%function [U_tot, u_out, v_out, w_out, p_out, q_out, r_out, pos_x_out, pos_y_out, pos_z_out, phi_out, theta_out, psi_out]  = otter(u, v, w, p, q, r, pos_x, pos_y, pos_z, phi, theta, psi ,F_1,F_2,alpha_1,alpha_2,n,mp,rp,V_c,beta_c)

% [xdot,U] = otter(x,n,mp,rp,V_c,beta_c) returns the speed U in m/s (optionally) 
% and the time derivative of the state vector: 

x = [u v w p q r pos_x pos_y pos_z phi theta psi]'; 
% for the Maritime Robotics Otter USV, see www.maritimerobotics.com. 
% The length of the USV is L = 2.0 m, while the state vector is defined as:
%
%  u:     surge velocity          (m/s)
%  v:     sway velocity           (m/s)
%  w:     heave velocity          (m/s)
%  p:     roll velocity           (rad/s)
%  q:     pitch velocity          (rad/s)
%  r:     yaw velocity            (rad/s)
%  x:     position in x direction (m)
%  y:     position in y direction (m)
%  z:     position in z direction (m)
%  phi:   roll angle              (rad)
%  theta: pitch angle             (rad)
%  psi:   yaw angle               (rad)
%
% The other inputs are:
%
% n = [ n(1) n(2) ]' where
%    n(1): propeller shaft speed, left (rad/s)
%    n(2): propeller shaft speed, right (rad/s)
%
% mp = payload mass (kg), maximum 45 kg
%  rp = [xp, yp, zp]' (m) is the location of the payload w.r.t. the CO
%  V_c:     current speed (m/s)
%  beta_c:  current direction (rad)
%
% See, ExOtter.m and demoOtterUSVHeadingControl.slx
%
% Author:    Thor I. Fossen
% Date:      2019-07-17
% Revisions: 2021-04-25 added call to new function crossFlowDrag.m
%            2021-06-21 Munk moment in yaw is neglected
%            2021-07-22 Added a new state for the trim moment
%            2021-12-17 New method Xudot = -addedMassSurge(m,L,rho) 

% Check of input and state dimensions
if (length(x) ~= 12),error('x vector must have dimension 12!'); end
if (length(n) ~= 2),error('n vector must have dimension 2!'); end

% trim: theta = -7.5 deg corresponds to 13.5 cm less height aft maximum load
trim_setpoint = 280;

% trim_setpoint is a step input, which is filtered using the state trim_moment
persistent trim_moment;

if isempty(trim_moment)
   trim_moment = 0;
end

% Main data
g   = 9.81;         % acceleration of gravity (m/s^2)
rho = 1025;         % density of water
L = 6.9;            % length (m)
B = 3.465;           % beam (m)
m = 775;           % mass (kg)
rg = [0 0 -0.1]'; % CG for hull only (m)
R44 = 0.4 * B;      % radii of gyrations (m)
R55 = 0.25 * L;
R66 = 0.25 * L;
T_yaw = 1;          % time constant in yaw (s)
Umax = 8 * 0.5144;  % max forward speed (m/s)

% Data for one pontoon
B_pont  = 0.696;     % beam of one pontoon (m)
y_pont  = 1.3395;    % distance from centerline to waterline area center (m)
Cw_pont = 0.75;     % waterline area coefficient (-)
Cb_pont = 0.4;      % block coefficient, computed from m = 55 kg


%%%%%%%%%%%%%%%%%%%%%%%%%%%%%%%%%%%%%%%%%%%%%%%%%%%%%%%%%%%%%%%%%%%%%%%%%%

% State and current variables
nu = x(1:6);                                % velocities
nu1 = x(1:3);                               % velocities
nu2 = x(4:6);                               % velocities
eta = x(7:12);                              % positions
U = sqrt(nu(1)^2 + nu(2)^2 + nu(3)^2);      % speed
u_c = V_c * cos(beta_c - eta(6));           % current surge velocity
v_c = V_c * sin(beta_c - eta(6));           % current sway velocity
nu_r = nu - [u_c v_c 0 0 0 0]';             % relative velocity vector

% Inertia dyadic, volume displacement and draft
nabla = (m+mp)/rho;                         % volume
T = nabla / (2 * Cb_pont * B_pont*L);       % draft
Ig_CG = m * diag([R44^2, R55^2, R66^2]);    % only hull in CG
rg = (m*rg + mp*rp)/(m+mp);           % CG location corrected for payload
Ig = Ig_CG - m * Smtrx(rg)^2 - mp * Smtrx(rp)^2;  % hull + payload in CO

% Experimental propeller data including lever arms
l1 = -y_pont;                           % lever arm, left propeller (m)
l2 = y_pont;                            % lever arm, right propeller (m)
k_pos = 0.02216/2;                      % Positive Bollard, one propeller 
k_neg = 0.01289/2;                      % Negative Bollard, one propeller 
n_max = 300.42; %sqrt((0.5*24.4 * g)/k_pos);    % maximum propeller rev. (rad/s)
n_min = -300.42; %-sqrt((0.5*13.6 * g)/k_neg);    % minimum propeller rev. (rad/s)

F_max = 1000;
F_min = -1000;


% MRB and CRB (Fossen 2021)
I3 = eye(3);
O3 = zeros(3,3);

MRB_CG = [ (m+mp) * I3  O3
           O3           Ig ];
CRB_CG = [ (m+mp) * Smtrx(nu2)         O3
           O3               -Smtrx(Ig*nu2)  ];

H = Hmtrx(rg);              % Transform MRB and CRB from the CG to the CO 
MRB = H' * MRB_CG * H;
CRB = H' * CRB_CG * H;

% Hydrodynamic added mass (best practise)
Xudot = -addedMassSurge(m,L,rho);   
Yvdot = -1.5 * m;
Zwdot = -1.0 * m;
Kpdot = -0.2 * Ig(1,1);
Mqdot = -0.8 * Ig(2,2);
Nrdot = -1.7 * Ig(3,3);

MA = -diag([Xudot, Yvdot, Zwdot, Kpdot, Mqdot, Nrdot]);   
CA  = m2c(MA, nu_r);
CA(6,1) = 0; % Assume that the Munk moment in yaw can be neglected
CA(6,2) = 0; % These terms, if nonzero, must be balanced by adding nonlinear damping

% System mass and Coriolis-centripetal matrices
M = MRB + MA;
C = CRB + CA;

% Hydrostatic quantities (Fossen 2021)
Aw_pont = Cw_pont * L * B_pont;    % waterline area, one pontoon 
I_T = 2 * (1/12)*L*B_pont^3 * (6*Cw_pont^3/((1+Cw_pont)*(1+2*Cw_pont)))...
    + 2 * Aw_pont * y_pont^2;
I_L = 0.8 * 2 * (1/12) * B_pont * L^3;
KB = (1/3)*(5*T/2 - 0.5*nabla/(L*B_pont) );
BM_T = I_T/nabla;       % BM values
BM_L = I_L/nabla;
KM_T = KB + BM_T;       % KM values
KM_L = KB + BM_L;
KG = T - rg(3);
GM_T = KM_T - KG;       % GM values
GM_L = KM_L - KG;

G33 = rho * g * (2 * Aw_pont);      % spring stiffness
G44 = rho * g *nabla * GM_T;
G55 = rho * g *nabla * GM_L;

G_CF = diag([0 0 G33 G44 G55 0]);   % spring stiffness matrix in the CF
LCF = -0.2;
H = Hmtrx([LCF 0 0]);               % transform G_CF from the CF to the CO 
G = H' * G_CF * H;

% Natural frequencies
w3 = sqrt( G33/M(3,3) );         
w4 = sqrt( G44/M(4,4) );
w5 = sqrt( G55/M(5,5) );

% Linear damping terms (hydrodynamic derivatives)
Xu = (-24.4 * g / Umax);           % specified using the maximum speed  
Yv = 0;
Zw = -2 * 0.3 *w3 * M(3,3);      % specified using relative damping factors
Kp = -2 * 0.2 *w4 * M(4,4);
Mq = -2 * 0.4 *w5 * M(5,5);
Nr = -M(6,6) / T_yaw;            % specified using the time constant in T_yaw

% Control forces and moments - with propeller revolution saturation 
% Thrust = zeros(2,1);
% for i = 1:1:2
%     if n(i) > n_max              % saturation, physical limits
%        n(i) = n_max; 
%     elseif n(i) < n_min
%        n(i) = n_min; 
%    end
%     
%    if n(i) > 0                          
%      Thrust(i) = k_pos * n(i)*abs(n(i));    % positive thrust (N) 
%    else
%      Thrust(i) = k_neg * n(i)*abs(n(i));    % negative thrust (N) 
%    end
% end

% % Control forces and moments
% tau = [Thrust(1) + Thrust(2) 0 0 0 0 -l1 * Thrust(1) - l2 * Thrust(2) ]';



% Control forces and moments - with propeller revolution saturation 
if F_1 > F_max              % saturation, physical limits
  F_1 = F_max; 
elseif F_1 < F_min
  F_1 = F_min; 
end
if F_2 > F_max              % saturation, physical limits
  F_2 = F_max; 
elseif F_1 < F_min
  F_2 = F_min; 
end



% Control forces and moments
tau = [F_1*cos(alpha_1)+F_2*cos(alpha_2) F_1*sin(alpha_1)+F_2*sin(alpha_2) 0 0 0 F_1*y_pont*cos(alpha_1)-F_2*y_pont*cos(alpha_2) ]';


% Linear damping using relative velocities + nonlinear yaw damping
Xh = Xu * nu_r(1);
Yh = Yv * nu_r(2); 
Zh = Zw * nu_r(3);
Kh = Kp * nu_r(4);
Mh = Mq * nu_r(5);
Nh = Nr * (1 + 10 * abs(nu_r(6))) * nu_r(6);

tau_damp = [Xh Yh Zh Kh Mh Nh]';

% Strip theory: cross-flow drag integrals for Yh and Nh
tau_crossflow = crossFlowDrag(L,B_pont,T,nu_r);

% Ballast
g_0 = [0 0 0 0 trim_moment 0]';

% Kinematics
J = eulerang(eta(4),eta(5),eta(6));

% Time derivative of the state vector - numerical integration; see ExOtter.m  
xdot = [ M \ ( tau + tau_damp + tau_crossflow - C * nu_r - nu - g_0)
         J * nu ];  
     
trim_moment = trim_moment + 0.05 * (trim_setpoint - trim_moment);





U_tot = U;
% u_out = xdot(1);
% v_out = xdot(2);
% w_out = xdot(3);
% p_out = xdot(4);
% q_out = xdot(5);
% r_out = xdot(6);
% pos_x_out = xdot(7);
% pos_y_out = xdot(8);
% pos_z_out = xdot(9); 
% phi_out = xdot(10);
% theta_out = xdot(11);
% psi_out = xdot(12);

end
